simulink model "ar_lht_hw_target"  (R2018a)
settings: Solver=VariableStepAuto  StartTime=0.0  StopTime=ts*4+(526+25)*4*T  RelTol=1e-3  EnableMultiTasking=on
PreLoadFcn:
  | currentDir  = pwd;
  | filesepIdx   = strfind(currentDir, filesep);
  | newDir = currentDir(1:filesepIdx(end)-7);
  | 
  | addpath([newDir, '\scripts']);
InitFcn:
  | setup;
  | pre_processing;
values from neighbouring files (symbols this model uses):
  deltaTheta = 1    [setup.m]
  fps = f/((height)*(width))    (= 138.282775879)    [setup.m]
  height = 1024    [setup.m]
  K = (maxTheta + deltaTheta)/R    (= 45)    [setup.m]
  maxRho = ceil(sqrt((height/2)^2+(width/2)^2))    [setup.m]
  maxTheta = 179    [setup.m]
  R = 4    [setup.m]
  T = 1/f    (= 6.89655172414e-09)    [setup.m]
  width = 1024    [setup.m]
libraries: xbsIndex_r4 x220, hdlsllib x6, visionhdlio x1, visionsources x1
(part 2 of 2)

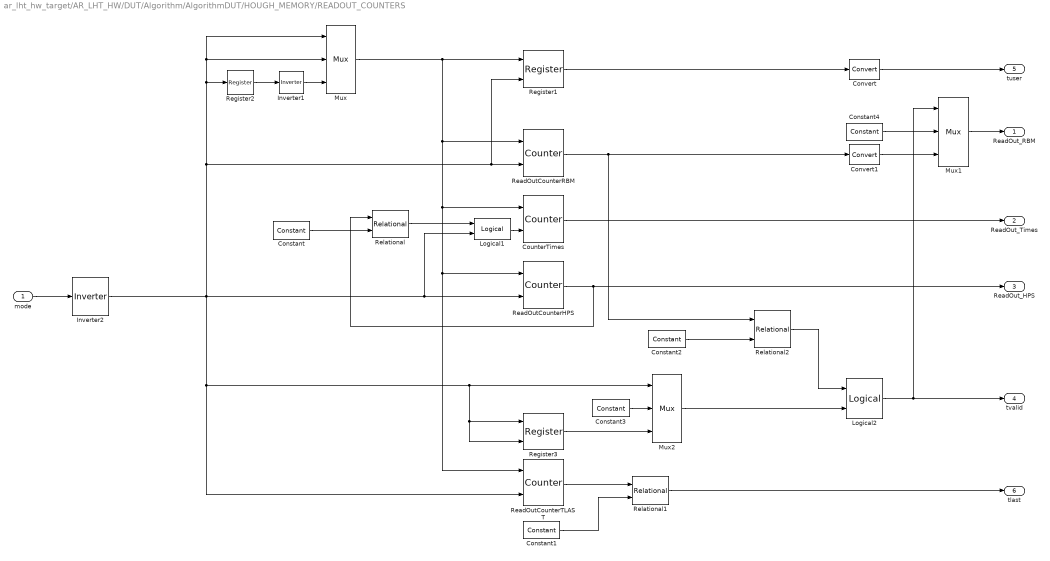
== system ar_lht_hw_target/AR_LHT_HW/DUT/Algorithm/AlgorithmDUT/HOUGH_MEMORY/READOUT_COUNTERS ==
  mode : Inport
  Constant : xbsIndex_r4/Constant  const=K*maxRho*2-2  gui_display_data_type=Fixed-point  arith_type=Unsigned  n_bits=ceil(log2(K*maxRho*2-2))  bin_pt=0  preci_type=Single  exp_width=8  frac_width=24  explicit_period=on  period=T  equ=P=C  opselect=C  inp2=PCIN>>17  opr=+  inp1=P  carry=CIN  dbl_ovrd=off  block_type=constant
  Constant1 : xbsIndex_r4/Constant  const=2*maxRho-1  gui_display_data_type=Fixed-point  arith_type=Unsigned  n_bits=ceil(log2(2*maxRho-1))  bin_pt=0  preci_type=Single  exp_width=8  frac_width=24  explicit_period=on  period=T  equ=P=C  opselect=C  inp2=PCIN>>17  opr=+  inp1=P  carry=CIN  dbl_ovrd=off  block_type=constant
  Constant2 : xbsIndex_r4/Constant  const=(maxTheta+deltaTheta)*maxRho*2-1  gui_display_data_type=Fixed-point  arith_type=Unsigned  n_bits=ceil(log2((maxTheta+deltaTheta)*maxRho*2-1))  bin_pt=0  preci_type=Single  exp_width=8  frac_width=24  explicit_period=on  period=T  equ=P=C  opselect=C  inp2=PCIN>>17  opr=+  inp1=P  carry=CIN  dbl_ovrd=off  block_type=constant
  Constant3 : xbsIndex_r4/Constant  const=0  gui_display_data_type=Boolean  arith_type=Boolean  n_bits=16  bin_pt=14  preci_type=Single  exp_width=8  frac_width=24  explicit_period=on  period=T  equ=P=C  opselect=C  inp2=PCIN>>17  opr=+  inp1=P  carry=CIN  dbl_ovrd=off  block_type=constant
  Constant4 : xbsIndex_r4/Constant  const=0  gui_display_data_type=Fixed-point  arith_type=Unsigned  n_bits=ceil(log2((maxTheta+deltaTheta)*maxRho*2-1))  bin_pt=0  preci_type=Single  exp_width=8  frac_width=24  explicit_period=on  period=T  equ=P=C  opselect=C  inp2=PCIN>>17  opr=+  inp1=P  carry=CIN  dbl_ovrd=off  block_type=constant
  Convert : xbsIndex_r4/Convert  gui_display_data_type=Fixed-point  arith_type=Unsigned  n_bits=1  bin_pt=0  float_type=Single  exp_bits=8  fraction_bits=24  quantization=Truncate  overflow=Wrap  en=off  latency=0  pipeline=off  dbl_ovrd=off  block_type=convert
  Convert1 : xbsIndex_r4/Convert  gui_display_data_type=Fixed-point  arith_type=Unsigned  n_bits=ceil(log2((maxTheta+deltaTheta)*maxRho*2-1))  bin_pt=0  float_type=Single  exp_bits=8  fraction_bits=24  quantization=Truncate  overflow=Wrap  en=off  latency=0  pipeline=off  dbl_ovrd=off  block_type=convert
  CounterTimes : xbsIndex_r4/Counter  cnt_type=Count Limited  cnt_to=R-1  operation=Up  start_count=0  cnt_by_val=1  arith_type=Unsigned  n_bits=ceil(log2(R))  bin_pt=0  load_pin=off  rst=on  en=on  explicit_period=on  period=T  use_behavioral_HDL=on  implementation=Fabric  dbl_ovrd=off  block_type=counter
  Inverter1 : xbsIndex_r4/Inverter  en=off  latency=0  dbl_ovrd=off  block_type=inv
  Inverter2 : xbsIndex_r4/Inverter  en=off  latency=0  dbl_ovrd=off  block_type=inv
  Logical1 : xbsIndex_r4/Logical  logical_function=AND  inputs=2  en=off  latency=0  precision=Full  arith_type=Unsigned  n_bits=16  bin_pt=0  align_bp=on  dbl_ovrd=off  block_type=logical
  Logical2 : xbsIndex_r4/Logical  logical_function=AND  inputs=2  en=off  latency=0  precision=Full  arith_type=Unsigned  n_bits=16  bin_pt=0  align_bp=on  dbl_ovrd=off  block_type=logical
  Mux : xbsIndex_r4/Mux  inputs=2  en=off  latency=0  precision=Full  arith_type=Unsigned  n_bits=16  bin_pt=14  quantization=Truncate  overflow=Wrap  dbl_ovrd=off  block_type=mux
  Mux1 : xbsIndex_r4/Mux  inputs=2  en=off  latency=0  precision=Full  arith_type=Unsigned  n_bits=16  bin_pt=14  quantization=Truncate  overflow=Wrap  dbl_ovrd=off  block_type=mux
  Mux2 : xbsIndex_r4/Mux  inputs=2  en=off  latency=0  precision=Full  arith_type=Unsigned  n_bits=16  bin_pt=14  quantization=Truncate  overflow=Wrap  dbl_ovrd=off  block_type=mux
  ReadOutCounterHPS : xbsIndex_r4/Counter  cnt_type=Count Limited  cnt_to=K*maxRho*2-1  operation=Up  start_count=0  cnt_by_val=1  arith_type=Unsigned  n_bits=ceil(log2(K*maxRho*2-1))  bin_pt=0  load_pin=off  rst=on  en=on  explicit_period=on  period=T  use_behavioral_HDL=on  implementation=Fabric  dbl_ovrd=off  block_type=counter
  ReadOutCounterRBM : xbsIndex_r4/Counter  cnt_type=Free Running  cnt_to=(maxTheta+deltaTheta)*maxRho*2-1  operation=Up  start_count=0  cnt_by_val=1  arith_type=Unsigned  n_bits=32  bin_pt=0  load_pin=off  rst=on  en=on  explicit_period=on  period=T  use_behavioral_HDL=on  implementation=Fabric  dbl_ovrd=off  block_type=counter
  ReadOutCounterTLAST : xbsIndex_r4/Counter  cnt_type=Count Limited  cnt_to=2*maxRho - 1  operation=Up  start_count=0  cnt_by_val=1  arith_type=Unsigned  n_bits=ceil(log2(2*maxRho-1))  bin_pt=0  load_pin=off  rst=on  en=on  explicit_period=on  period=T  use_behavioral_HDL=on  implementation=Fabric  dbl_ovrd=off  block_type=counter
  Register1 : xbsIndex_r4/Register  init=0  rst=off  en=on  dbl_ovrd=off  block_type=register
  Register2 : xbsIndex_r4/Register  init=0  rst=off  en=off  dbl_ovrd=off  block_type=register
  Register3 : xbsIndex_r4/Register  init=0  rst=off  en=on  dbl_ovrd=off  block_type=register
  Relational : xbsIndex_r4/Relational  mode=a=b  op_type=Bool  en=off  latency=1  dbl_ovrd=off  block_type=relational
  Relational1 : xbsIndex_r4/Relational  mode=a=b  op_type=Bool  en=off  latency=0  dbl_ovrd=off  block_type=relational
  Relational2 : xbsIndex_r4/Relational  mode=a<=b  op_type=Bool  en=off  latency=0  dbl_ovrd=off  block_type=relational
  ReadOut_RBM : Outport
  ReadOut_Times : Outport  Port=2
  ReadOut_HPS : Outport  Port=3
  tvalid : Outport  Port=4
  tuser : Outport  Port=5
  tlast : Outport  Port=6
  wires:
  Relational/1 -> Logical1/1
  Logical1/1 -> CounterTimes/2
  Constant/1 -> Relational/2
  ReadOutCounterRBM/1 -> Relational2/1, Convert1/1
  CounterTimes/1 -> ReadOut_Times/1
  ReadOutCounterHPS/1 -> ReadOut_HPS/1, Relational/1
  mode/1 -> Inverter2/1
  Register2/1 -> Inverter1/1
  Inverter1/1 -> Mux/3
  Relational1/1 -> tlast/1
  ReadOutCounterTLAST/1 -> Relational1/1
  Constant1/1 -> Relational1/2
  Convert/1 -> tuser/1
  Constant2/1 -> Relational2/2
  Mux/1 -> Register1/1, ReadOutCounterTLAST/1, ReadOutCounterHPS/1, CounterTimes/1, ReadOutCounterRBM/1
  Register1/1 -> Convert/1
  Relational2/1 -> Logical2/1
  Register3/1 -> Mux2/3
  Mux2/1 -> Logical2/2
  Inverter2/1 -> ReadOutCounterTLAST/2, Register3/2, Register3/1, Mux2/1, Logical1/2, ReadOutCounterHPS/2, Register1/2, ReadOutCounterRBM/2, Mux/1, Mux/2, Register2/1
  Constant3/1 -> Mux2/2
  Mux1/1 -> ReadOut_RBM/1
  Convert1/1 -> Mux1/3
  Constant4/1 -> Mux1/2
  Logical2/1 -> tvalid/1, Mux1/1

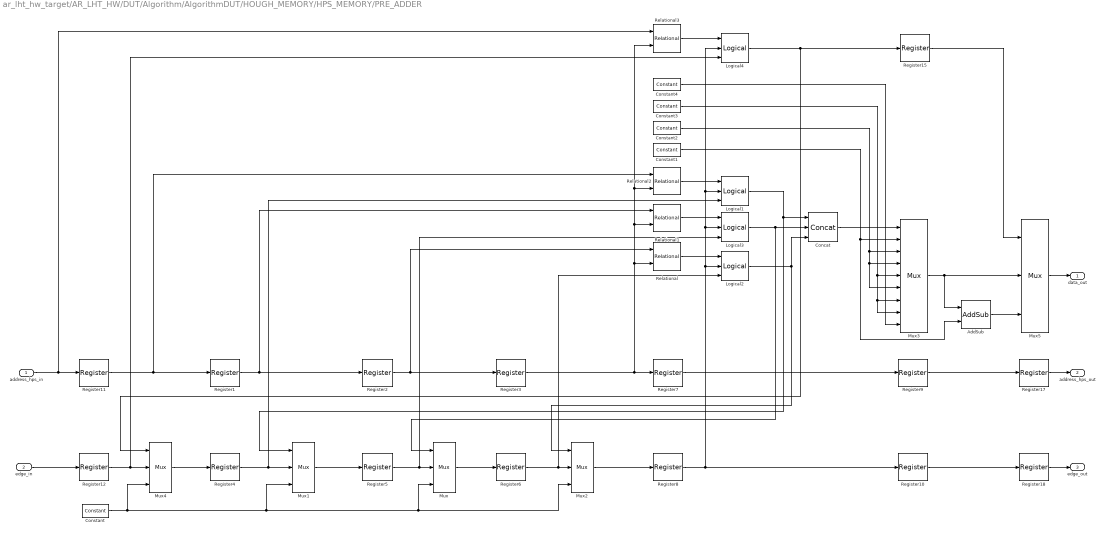
== system ar_lht_hw_target/AR_LHT_HW/DUT/Algorithm/AlgorithmDUT/HOUGH_MEMORY/HPS_MEMORY/PRE_ADDER ==
  address_hps_in : Inport
  edge_in : Inport  Port=2
  AddSub : xbsIndex_r4/AddSub  mode=Addition  use_carryin=off  use_carryout=off  en=off  latency=0  precision=User Defined  arith_type=Unsigned  n_bits=3  bin_pt=0  quantization=Truncate  overflow=Wrap  use_behavioral_HDL=off  hw_selection=Fabric  pipelined=off  dbl_ovrd=off  block_type=addsub
  Concat : xbsIndex_r4/Concat  num_inputs=3  dbl_ovrd=off  block_type=concat
  Constant : xbsIndex_r4/Constant  const=0  gui_display_data_type=Boolean  arith_type=Boolean  n_bits=16  bin_pt=14  preci_type=Single  exp_width=8  frac_width=24  explicit_period=on  period=T  equ=P=C  opselect=C  inp2=PCIN>>17  opr=+  inp1=P  carry=CIN  dbl_ovrd=off  block_type=constant
  Constant1 : xbsIndex_r4/Constant  const=1  gui_display_data_type=Fixed-point  arith_type=Unsigned  n_bits=3  bin_pt=0  preci_type=Single  exp_width=8  frac_width=24  explicit_period=on  period=T  equ=P=C  opselect=C  inp2=PCIN>>17  opr=+  inp1=P  carry=CIN  dbl_ovrd=off  block_type=constant
  Constant2 : xbsIndex_r4/Constant  const=2  gui_display_data_type=Fixed-point  arith_type=Unsigned  n_bits=3  bin_pt=0  preci_type=Single  exp_width=8  frac_width=24  explicit_period=on  period=T  equ=P=C  opselect=C  inp2=PCIN>>17  opr=+  inp1=P  carry=CIN  dbl_ovrd=off  block_type=constant
  Constant3 : xbsIndex_r4/Constant  const=3  gui_display_data_type=Fixed-point  arith_type=Unsigned  n_bits=3  bin_pt=0  preci_type=Single  exp_width=8  frac_width=24  explicit_period=on  period=T  equ=P=C  opselect=C  inp2=PCIN>>17  opr=+  inp1=P  carry=CIN  dbl_ovrd=off  block_type=constant
  Constant4 : xbsIndex_r4/Constant  const=4  gui_display_data_type=Fixed-point  arith_type=Unsigned  n_bits=3  bin_pt=0  preci_type=Single  exp_width=8  frac_width=24  explicit_period=on  period=T  equ=P=C  opselect=C  inp2=PCIN>>17  opr=+  inp1=P  carry=CIN  dbl_ovrd=off  block_type=constant
  Logical{1..4} (4 alike) : xbsIndex_r4/Logical  logical_function=AND  inputs=3  en=off  latency=0  precision=Full  arith_type=Unsigned  n_bits=16  bin_pt=0  align_bp=on  dbl_ovrd=off  block_type=logical
  Mux{,1..2,4} (4 alike) : xbsIndex_r4/Mux  inputs=2  en=off  latency=0  precision=Full  arith_type=Unsigned  n_bits=16  bin_pt=14  quantization=Truncate  overflow=Wrap  dbl_ovrd=off  block_type=mux
  Mux3 : xbsIndex_r4/Mux  inputs=8  en=off  latency=1  precision=Full  arith_type=Unsigned  n_bits=16  bin_pt=14  quantization=Truncate  overflow=Wrap  dbl_ovrd=off  block_type=mux
  Mux5 : xbsIndex_r4/Mux  inputs=2  en=off  latency=1  precision=Full  arith_type=Unsigned  n_bits=16  bin_pt=14  quantization=Truncate  overflow=Wrap  dbl_ovrd=off  block_type=mux
  Register{1..12,15,17..18} (15 alike) : xbsIndex_r4/Register  init=0  rst=off  en=off  dbl_ovrd=off  block_type=register
  Relational{,1..3} (4 alike) : xbsIndex_r4/Relational  mode=a=b  op_type=Bool  en=off  latency=1  dbl_ovrd=off  block_type=relational
  data_out : Outport
  address_hps_out : Outport  Port=2
  edge_out : Outport  Port=3
  wires:
  address_hps_in/1 -> Relational3/1, Register11/1
  Register1/1 -> Register2/1, Relational1/1
  Register2/1 -> Register3/1, Relational/1
  Register3/1 -> Register7/1, Relational3/2, Relational2/2, Relational1/2, Relational/2
  Register7/1 -> Register9/1
  Register8/1 -> Logical3/2, Logical4/2, Logical1/2, Logical2/2, Register10/1
  Mux/1 -> Register6/1
  Mux1/1 -> Register5/1
  Register4/1 -> Logical1/3, Mux1/2
  edge_in/1 -> Register12/1
  Concat/1 -> Mux3/1
  Register6/1 -> Logical2/3, Mux2/2
  Mux2/1 -> Register8/1
  Constant/1 -> Mux4/3, Mux/3, Mux2/3, Mux1/3
  Constant1/1 -> AddSub/2, Mux3/2
  Constant2/1 -> Mux3/6, Mux3/4, Mux3/3
  Constant3/1 -> Mux3/7, Mux3/8, Mux3/5
  Constant4/1 -> Mux3/9
  Logical1/1 -> Mux1/1, Concat/1
  Relational2/1 -> Logical1/1
  Logical3/1 -> Mux/1, Concat/2
  Relational1/1 -> Logical3/1
  Relational/1 -> Logical2/1
  Logical2/1 -> Concat/3, Mux2/1
  Register5/1 -> Logical3/3, Mux/2
  Register11/1 -> Register1/1, Relational2/1
  Register12/1 -> Mux4/2, Logical4/3
  Mux4/1 -> Register4/1
  Relational3/1 -> Logical4/1
  AddSub/1 -> Mux5/3
  Mux3/1 -> Mux5/2, AddSub/1
  Logical4/1 -> Mux4/1, Register15/1
  Register15/1 -> Mux5/1
  Mux5/1 -> data_out/1
  Register9/1 -> Register17/1
  Register10/1 -> Register18/1
  Register18/1 -> edge_out/1
  Register17/1 -> address_hps_out/1

== system ar_lht_hw_target/AR_LHT_HW/DUT/Algorithm/AlgorithmDUT/HOUGH_MEMORY/HPS_MEMORY/Registers ==
  In1 : Inport
  Register1 : xbsIndex_r4/Register  init=0  rst=off  en=off  dbl_ovrd=off  block_type=register
  Register5 : xbsIndex_r4/Register  init=0  rst=off  en=off  dbl_ovrd=off  block_type=register
  Register7 : xbsIndex_r4/Register  init=0  rst=off  en=off  dbl_ovrd=off  block_type=register
  Out1 : Outport
  wires:
  Register5/1 -> Register7/1
  In1/1 -> Register1/1
  Register7/1 -> Out1/1
  Register1/1 -> Register5/1

== system ar_lht_hw_target/AR_LHT_HW/DUT/Algorithm/AlgorithmDUT/HOUGH_MEMORY/HPS_MEMORY/Registers1 ==
  In1 : Inport
  Register1 : xbsIndex_r4/Register  init=0  rst=off  en=off  dbl_ovrd=off  block_type=register
  Register5 : xbsIndex_r4/Register  init=0  rst=off  en=off  dbl_ovrd=off  block_type=register
  Register7 : xbsIndex_r4/Register  init=0  rst=off  en=off  dbl_ovrd=off  block_type=register
  Out1 : Outport
  wires:
  Register1/1 -> Register5/1
  Register7/1 -> Out1/1
  In1/1 -> Register1/1
  Register5/1 -> Register7/1

== system ar_lht_hw_target/AR_LHT_HW/DUT/Algorithm/AlgorithmDUT/HOUGH_MEMORY/HPS_MEMORY/Registers2 ==
  In1 : Inport
  Register1 : xbsIndex_r4/Register  init=0  rst=off  en=off  dbl_ovrd=off  block_type=register
  Register5 : xbsIndex_r4/Register  init=0  rst=off  en=off  dbl_ovrd=off  block_type=register
  Register7 : xbsIndex_r4/Register  init=0  rst=off  en=off  dbl_ovrd=off  block_type=register
  Out1 : Outport
  wires:
  Register5/1 -> Register7/1
  In1/1 -> Register1/1
  Register7/1 -> Out1/1
  Register1/1 -> Register5/1

== system ar_lht_hw_target/AR_LHT_HW/DUT/Algorithm/AlgorithmDUT/HOUGH_MEMORY/HPS_MEMORY/Registers3 ==
  In1 : Inport
  Register1 : xbsIndex_r4/Register  init=0  rst=off  en=off  dbl_ovrd=off  block_type=register
  Register5 : xbsIndex_r4/Register  init=0  rst=off  en=off  dbl_ovrd=off  block_type=register
  Register7 : xbsIndex_r4/Register  init=0  rst=off  en=off  dbl_ovrd=off  block_type=register
  Out1 : Outport
  wires:
  Register1/1 -> Register5/1
  Register7/1 -> Out1/1
  In1/1 -> Register1/1
  Register5/1 -> Register7/1

== system ar_lht_hw_target/AR_LHT_HW/DUT/Algorithm/AlgorithmDUT/HOUGH_MEMORY/HPS_MEMORY/Registers4 ==
  In1 : Inport
  Register1 : xbsIndex_r4/Register  init=0  rst=off  en=off  dbl_ovrd=off  block_type=register
  Register5 : xbsIndex_r4/Register  init=0  rst=off  en=off  dbl_ovrd=off  block_type=register
  Register7 : xbsIndex_r4/Register  init=0  rst=off  en=off  dbl_ovrd=off  block_type=register
  Out1 : Outport
  wires:
  Register5/1 -> Register7/1
  In1/1 -> Register1/1
  Register7/1 -> Out1/1
  Register1/1 -> Register5/1
